simulink model "IceStorage_FHNW"  (R2018b)
settings: Solver=ode23  StartTime=-122*24*3600  StopTime=(365+181)*24*3600  EnableMultiTasking=on
StartFcn:
  | ticID_VsIceSTsim = tic;
StopFcn:
  | toc(ticID_VsIceSTsim)
undefined symbols (not defined in the file or in its folder): A, B, C, Davies, Dd, Hay
libraries: carnot x43, simulink x3, carsys x1
(part 1 of 2)
settings Model: SimulationMode=accelerator  Creator=ralf.dott  LastModifiedBy=drhf
settings DataIOCC: SaveFormat=Array  SignalLoggingSaveFormat=ModelDataLogs  SaveOutput=off  SignalLogging=off  DSMLogging=off  SaveTime=off
settings OptimizationCC: ExpressionDepthLimit=2147483647  LifeSpan=inf
settings DebuggingCC: UnderspecifiedInitializationDetection=Classic  MergeDetectMultiDrivingBlocksExec=none  SolverPrmCheckMsg=warning  FcnCallInpInsideContextMsg=warning  StateNameClashWarn=warning  SFUnexpectedBacktrackingDiag=warning  SFNoUnconditionalDefaultTransitionDiag=warning  SFExecutionAtInitializationDiag=none
settings HardwareCC: ProdBitPerPointer=32  ProdBitPerSizeT=32  ProdBitPerPtrDiffT=32  ProdLargestAtomicFloat=None  ProdIntDivRoundTo=Undefined  ProdEndianess=Unspecified  ProdWordSize=32  ProdHWDeviceType=32-bit Generic
settings ModelReferenceCC: PropagateSignalLabelsOutOfModel=off
settings SFSimCC: SimUseLocalCustomCode=off
settings RTWCC: RTWUseLocalCustomCode=off
settings CodeAppCC: StateflowObjectComments=on
settings GRTTargetCC: TargetLangStandard=C89/C90 (ANSI)  GeneratePreprocessorConditionals=Disable all  CombineOutputUpdateFcns=off  GRTInterface=on
settings ConfigComp: CovMetricSettings=dw  CovHtmlReporting=on  CovSaveCumulativeToWorkspaceVar=on  CovSaveSingleToWorkspaceVar=on  CovExternalEMLEnable=off

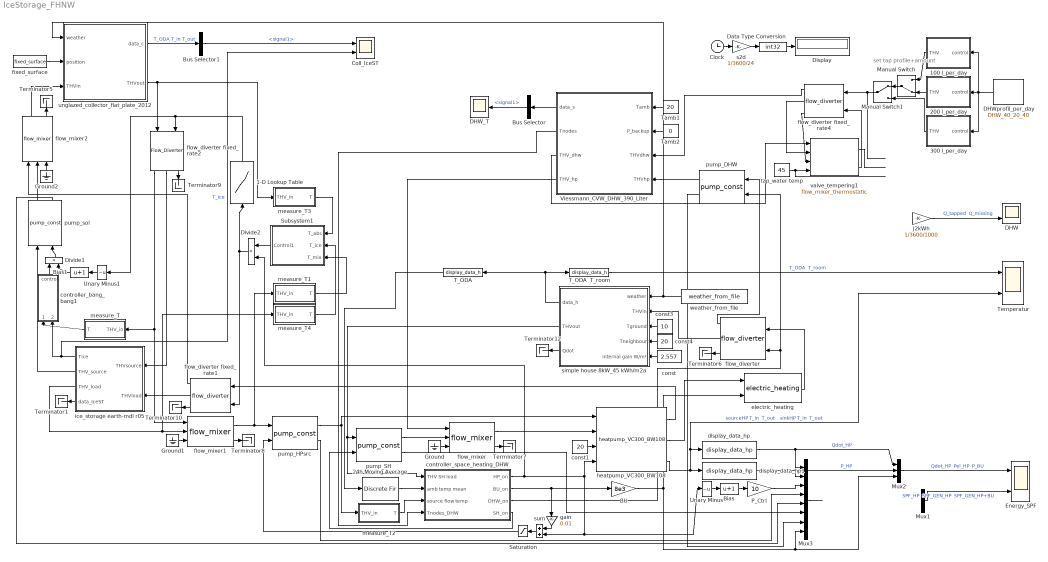
== system IceStorage_FHNW ==
  note: set tap
      | profile+amount
  1-D Lookup Table : Lookup_n-D  NumberOfTableDimensions=1  BreakpointsForDimension1=[-10, 0, eps, 10]  Table=[0, 0, 1, 1]  RndMeth=Simplest  InputSameDT=on
  100 l_per_day : Subsystem  mask(water tap){T=10, Tamp=3, dshift=-137, mdot=100/1800, fluid_id=water, mix=0, dia=0.013, p=2e5}
      mask prompts: T "mean temperature [degree centigrade]"; Tamp "amplitude of the sine [k]"; dshift "phase shift of the sine in [days]"; mdot "massflow [kg/s]"; fluid_id "fluid"; mix "percentage of fluid mix [0..1]"; dia "diameter at outlet [m]"; p "system pressure [Pa]"
      mask help:
      | The block models a tap, that produces a constant massflow of a fluid at given times.
      | control = 1 is full massflow, control = 0 is no massflow.
      | The temperature is a sine wave according to:
      |
      | T(out) = T(mean) + T(amplitude) * sin( 2*PI*(SimulationDay + DayPhaseShift) / 365 )
      mask init:
      | mdot = max(0, mdot);
      | mix = min(1, max(0, mix));
      | dia = max(0.001, dia);
      | p = max(p, 1e5);
      mask Help: eval('htmlhelp (''chap_4_2w.htm#water_tap'')')
      mask TypeOptions fluid_id: water | air | cotton_oil | silicone_oil | water_glycol_mix
      mask Display: plot(-10,10,90,90,[44,67,67,45,45,40,40,44],[80,80,72,72,60,60,76,80],[60,45],[90,90],[53,53],[80,90],[24,29,70,75,24],[30,10,10,30,30],[42,42],[32,58],[46,44],[34,54],[38,40],[34,56])
  200 l_per_day : Subsystem  mask(water tap){T=10, Tamp=3, dshift=-137, mdot=200/1800, fluid_id=water, mix=0, dia=0.013, p=2e5}
      mask prompts: T "mean temperature [degree centigrade]"; Tamp "amplitude of the sine [k]"; dshift "phase shift of the sine in [days]"; mdot "massflow [kg/s]"; fluid_id "fluid"; mix "percentage of fluid mix [0..1]"; dia "diameter at outlet [m]"; p "system pressure [Pa]"
      mask help:
      | The block models a tap, that produces a constant massflow of a fluid at given times.
      | control = 1 is full massflow, control = 0 is no massflow.
      | The temperature is a sine wave according to:
      |
      | T(out) = T(mean) + T(amplitude) * sin( 2*PI*(SimulationDay + DayPhaseShift) / 365 )
      mask init:
      | mdot = max(0, mdot);
      | mix = min(1, max(0, mix));
      | dia = max(0.001, dia);
      | p = max(p, 1e5);
      mask Help: eval('htmlhelp (''chap_4_2w.htm#water_tap'')')
      mask TypeOptions fluid_id: water | air | cotton_oil | silicone_oil | water_glycol_mix
      mask Display: plot(-10,10,90,90,[44,67,67,45,45,40,40,44],[80,80,72,72,60,60,76,80],[60,45],[90,90],[53,53],[80,90],[24,29,70,75,24],[30,10,10,30,30],[42,42],[32,58],[46,44],[34,54],[38,40],[34,56])
  24h Moving Average : DiscreteFir  Coefficients=ones(1,24)*(1/24)  SampleTime=3600  RndMeth=Nearest
  300 l_per_day : Subsystem  mask(water tap){T=10, Tamp=3, dshift=-137, mdot=300/1800, fluid_id=water, mix=0, dia=0.013, p=2e5}
      mask prompts: T "mean temperature [degree centigrade]"; Tamp "amplitude of the sine [k]"; dshift "phase shift of the sine in [days]"; mdot "massflow [kg/s]"; fluid_id "fluid"; mix "percentage of fluid mix [0..1]"; dia "diameter at outlet [m]"; p "system pressure [Pa]"
      mask help:
      | The block models a tap, that produces a constant massflow of a fluid at given times.
      | control = 1 is full massflow, control = 0 is no massflow.
      | The temperature is a sine wave according to:
      |
      | T(out) = T(mean) + T(amplitude) * sin( 2*PI*(SimulationDay + DayPhaseShift) / 365 )
      mask init:
      | mdot = max(0, mdot);
      | mix = min(1, max(0, mix));
      | dia = max(0.001, dia);
      | p = max(p, 1e5);
      mask Help: eval('htmlhelp (''chap_4_2w.htm#water_tap'')')
      mask TypeOptions fluid_id: water | air | cotton_oil | silicone_oil | water_glycol_mix
      mask Display: plot(-10,10,90,90,[44,67,67,45,45,40,40,44],[80,80,72,72,60,60,76,80],[60,45],[90,90],[53,53],[80,90],[24,29,70,75,24],[30,10,10,30,30],[42,42],[32,58],[46,44],[34,54],[38,40],[34,56])
  BU : Gain  Gain=8e3
  Bias : Bias  Bias=1
  Bias1 : Bias  Bias=1
  Bus Selector : BusSelector  OutputSignals=signal1
  Bus Selector1 : BusSelector  OutputSignals=signal1
  Clock : Clock
      settings: Decimation=3600
  Coll_IceST : Scope  NumInputPorts=2
  DHW : Scope  NumInputPorts=2
  DHW_T : Scope
  DHWprofil_per_day : carnot/loads/DHW_40_20_40  period=24*3600  rep_seq_t=[7 12 19]*3600  rep_seq_d=[0.2 0.1 0.2]*3600  rep_seq_y=[1 1 1]
      settings: SourceProductName=Carnot
  Data Type Conversion : DataTypeConversion  OutDataTypeStr=int32
  Display : Display
  Divide1 : Product  Inputs=**
  Divide2 : Product  Inputs=**
  Energy_SPF : Scope  NumInputPorts=2
  Ground : Ground
  Ground1 : Ground
  Ground2 : Ground
  J2kWh : Gain  Gain=1/3600/1000
  Manual Switch : ManualSwitch  CurrentSetting=0
  Manual Switch1 : ManualSwitch
  Mux1 : Mux  Inputs=3
  Mux2 : Mux  Inputs=3
  Mux3 : Mux  Inputs=8
  P_Ctrl : Gain  Gain=10
  Saturation : Saturate  UpperLimit=1  LowerLimit=0
  Subsystem1 : Subsystem
  T_ODA : carnot/outputs/display_data_h  a01=on  a02=off  a03=off  a04=off  a05=off  a06=off
      settings: SourceProductName=Carnot
  T_ODA  T_room : carnot/outputs/display_data_h  a01=on  a02=on  a03=off  a04=off  a05=off  a06=off
      settings: SourceProductName=Carnot
  Tamb1 : Constant  Value=20
  Tamb2 : Constant  Value=0
  Temperatur : Scope  NumInputPorts=2
  Terminator{1,5..10,12} (8 alike) : Terminator
  Unary Minus : UnaryMinus
  Unary Minus1 : UnaryMinus
  Viessmann_CVW_DHW_390_Liter : Subsystem  mask(storage with heat exchangers){diameter=0.65, vol=0.395, pos=standing cylinder, heatloss=2.34/(pi*0.65*(0.41/(pi*(0.65/2)^2))), hlossbot=0.34/(pi*(0.65/2)^2), hlosstop=2.34/(pi*0.65*(0.41/(pi*(0.65/2)^2))), axialcond=1.21, tinitial=45}
      mask prompts: diameter "diameter [m]"; vol "volume in [m³]"; pos "position"; heatloss "heat loss coefficient wall in [W/(m²*K)]"; hlossbot "heat loss coefficient bottom [W/(m²*K)]"; hlosstop "heat loss coefficient top [W/(m²*K)]"; axialcond "effective axial conductivity in [W/(m*K)]"; tinitial "initial temperature in [degree centigrade]"
      mask help:
      | Parameterized for the Vitocell 100-V type CVB, 300 liter domestic hot water cylinder.
      | Test data from itw 04STO103 06aug2004
      | Temperature sensor position (relative height)
      |     Solar: 0.04
      |     Backup heating DHW: 0.62
      mask Help: eval('man(''storage_multiport'')')
      mask TypeOptions pos: lying cylinder | standing cylinder
      mask Display: plot(0,0,100,100,[36,36,40,50,54,54,50,40,36],[90,50,45,45,50,90,93,93,90],[36,51,40,51,36],[74,74,79,85,85],[36,51,44,51,36],[54,54,56,58,58])
  const : Constant  Value=2.557
  const1 : Constant  Value=20
  const3 : Constant  Value=10
  const4 : Constant  Value=20
  controller_bang_bang1 : Subsystem  AncestorBlock=carnot/control/controller_bang_bang  mask(bang bang controler){deltaTon=6, deltaToff=2, Tmax=20}
      mask prompts: deltaTon "deltaT-on [K]"; deltaToff "deltaT-off [K]"; Tmax "maximum temperature Tcold [degree centigrade]"
      mask help:
      | Hysteresis controller for thermal systems. Output is set to zero if Thot or Tcold is bigger than Tmax.
      | deltaT = Thot - Tcold
      mask Help: eval('man (''bang_bang_controller'')')
      mask Display: plot(-30,0,150,100,[70,100,40,10,70,70,10,10],[50,80,80,50,50,20,20,50],[100,70],[50,20],[20,50,50,20,20],[40,40,30,30,40],[62,62,62,61,59,58,58,60],[42,41,39,38,38,40,42,43],[61,62,62,61,60,59,58,58,58,59],[32,31,30,28,27,28,28,30,31,32])
  controller_space_heating_DHW : Subsystem  mask(controller depending on ambient temperature and return temperature){Temin=-10, Ta_deltaHK=20, deltaHK=0, offsetTset=[0 0], HG=14, tmodi=[0 6 6 11 11 12 12 18 18 19 19 22 22 24]*3600, gammamodi=[1 1 1 1 1 1 1 1 0 0 1 1 1 1]*100   %100=spaceheating 200=DHW, deltaTRset=[1 -1], deltaTSset=[1 -1], Tiset=[20 20], tN=[22 6], m=1.1, TaD=-8, TD=[33 28], returnCTRLon=on, T_DHW=50, T_DHW_max=95, pos_DHW=0.4}
      mask prompts: Temin "min source input temperature [°C]"; Ta_deltaHK "ambient temperature for gradient modification [°C]"; deltaHK "elevation of feetpoint temperature [K] (for gradient modification)"; offsetTset "offset heating curve [TRset TSset]"; HG "heating limit"; tmodi "time values for schedule modi"; gammamodi "modi values for schedule modi"; deltaTRset "hysteresis TR lower and upper band [K]"; deltaTSset "hysteresis TS lower and upper band [K]"; Tiset "room temperature setpoint [day night] [°C]"; tN "night set back [starttime stoptime] [h]"; m "coefficient of heating surfaces [1...1.3]"; TaD "ambient temperature case of design [°C]"; TD "[supply return] temperature case of design [°C]"; returnCTRLon "control return temperature and connect return to "THV SH load" (off = flow temp.)"; T_DHW "domestic hot water temperature [°C]"; T_DHW_max "maximum domestic hot water temperature [°C]"; pos_DHW "storage height of control temp. sensor 0..1 (0=bottom 1=top)"
      mask help:
      | Calculating the heating curve dependent on return temperature and ambient temperature on basis of design temperature of return and supply as well as ambient design temperature with hysteresis.
      | The on SIA 384/2 based calculation of the heating curve can be modified to tune the gradient and give an offset.
      | With a time schedule the primacy of making warm water can be defined and a night set back can be destined.
      mask init:
      | if  tN(1)>24;
      |     error('unaccepted time values are set for night set back in block controller');
      | end;
      | if  tN(1)<0;
      |     error('unaccepted time values are set for night set back in block controller');
      | end;
      | if  tN(2)>24;
      |     error('unaccepted time values are set for night set back in block controller');
      | end;
      | if  tN(2)<0;
      |     error('unaccepted time values are set for night set back in block controller');
      | end;
      | if  m>2;
      |     error('unaccepted value for coefficient of heating surface in block controller');
      | end;
      | if  m>1.3;
      |     error('unaccepted value for coefficient of heating surface in block controller');
      | end;
      | if  m>1.3;
      |     error('unaccepted value for coefficient of heating surface in block controller');
      | end;
      | if  m<1;
      |     error('unaccepted value for coefficient of heating surface in block controller');
      | end;
      mask Help:
      | created   20.12.01 FHBB Institut of Energy suw
      | updated  18.01.02 FHBB Institut of Energy suw / night setback correction
      | updated  21.01.02 FHBB Institut of Energy suw / calculating TSset
      |                                                                            / using schedules
      |                                                                            / error criteria
      |                                                                            / heating limit HG
      |                                                                            / heating curve offset
      mask Display: plot(-100,-40,130,60, [70,10,70,70,10,10], [50,50,50,20,20,50], [20,50,50,20,20],[40,40,30,30,40], [62,62,62,61,59,58,58,60], [42,41,39,38,38,40,42,43], [61,62,62,61,60,59,58,58,58,59], [32,31,30,28,27,28,28,30,31,32])
  display_data_hp : carnot/outputs/display_data_hp  a1=off  a2=off  a3=off  a4=off  a5=off  a6=off  a7=off  a8=on  a9=off
      settings: SourceProductName=Carnot
  display_data_hp1 : carnot/outputs/display_data_hp  a1=off  a2=off  a3=off  a4=off  a5=off  a6=off  a7=off  a8=off  a9=on
      settings: SourceProductName=Carnot
  electric_heating : carnot/heat_source/electric_heating
      settings: SourceProductName=Carnot
  fixed_surface : carnot/weather/fixed_surface  colangle=40  colazi=0  colrot=0
      settings: SourceProductName=Carnot
  flow_diverter : carnot/hydraulics/flow_diverter  t=1
      settings: SourceProductName=Carnot
  flow_diverter fixed_rate1 : carnot/hydraulics/flow_diverter  t=5
      settings: SourceProductName=Carnot
  flow_diverter fixed_rate2 : carnot/hydraulics/Flow_Diverter  t=5
      settings: SourceProductName=Carnot
  flow_diverter fixed_rate4 : carnot/hydraulics/flow_diverter  t=5
      settings: SourceProductName=Carnot
  flow_mixer : carnot/hydraulics/flow_mixer  t=1
      settings: SourceProductName=Carnot
  flow_mixer1 : carnot/hydraulics/flow_mixer  t=1
      settings: SourceProductName=Carnot
  flow_mixer2 : carnot/hydraulics/flow_mixer  t=1
      settings: SourceProductName=Carnot
  gain : Gain  Gain=0.01
  heatpump_VC300_BW108 : carsys/heat_source/heatpump_VC300_BW108  caph=8*4e3  capc=4*4e3  dp=[100 1e4]  UA=5  Tcin=[0 15]  Thout=[35 55]  Qdoth=[7850 7100; 11500 10300]  Qdotc=[6300 4600; 9950 7850]  Pel=[1720 2690; 1670 2600]
      settings: SourceProductName=Carnot
  ice_storage earth-mdl r05 : Subsystem  mask(simple water storage){vol=10, l_solar=195, l_hp=7*50, f_ice=0, t_ini=15, z=3.32-0.12, h=2.3, dearth=0.5, Tmeanoutside=11, deltathetae=9.3, Tmeaninside=5, deltathetai=15, tshift=319, cond_ground=2, cp_ground=800, rho_ground=2500}
      mask prompts: vol "volume [m³]"; l_solar "length of solar heat exchanger [m]"; l_hp "length of HP heat exchanger [m]"; f_ice "Initial fraction of ice (0..1)"; t_ini "Initial Temperatur (only if fraction ice = 0) [°C]"; z "depth of baseplate from upper surface [m]"; h "height of ice storage [m]"; dearth "thickness of surrounding earth layer [m]"; Tmeanoutside "mean outside temperature over one year [°C]"; deltathetae "amplitude of monthly outside temperatures [°C]"; Tmeaninside "mean inside temperature over one year [°C]"; deltathetai "amplitude of monthly mean inside temperature [°C]"; tshift "time shift where external temperature sine-curve shows a minimum [h]"; cond_ground "conductivity of ground [W/(m*K)]"; cp_ground "capacity of ground [J/(kg*K)]"; rho_ground "density of ground [kg/m^3]"
      mask help: multinode water storage
      mask init:
      | f_ice = min(1, max(0, f_ice));
      | h_ini = (1-f_ice)*335e3;
      | if f_ice == 0 
      |     h_ini = h_ini + 4182*t_ini;
      | end
      | %Durchmesser Eisspeicher [m]
      | D_tank = 2.7;
      | %Höhe Eisspeicher [m]
      | h_tank = 2.3;
      | %Grundfläche [m^2]
      | A = pi*(D_tank/2.)^2;
      | %Umfang [m]
      | P = D_tank*pi;
      | %charakteristisches Bodenmass [m]
      | B = A/(0.5*P);
      | %Wärmewiderstand Boden & Wand [m^2*K/W]
      | Rbtot = 0.12/1.330;
      | Rwtot = 0.1/1.330;
      | %Wanddicke [m]
      | w = 0.1;
      | %wirksame Dicke Boden & Wand [m]
      | dt = w + cond_ground*Rbtot;
      | dw = cond_ground*Rwtot;
      | %abstand der mitte der wandfläche zur oberfläche [m]
      | ztilde = z-(0.5*h);
      | %anzahl stunden pro jahr
      | t0 = 8760;
      | %thermische eindringtiefe
      | delta_grd = sqrt((t0*3600*cond_ground)/(pi*rho_ground*cp_ground));
      | 
      | %U-Wert Erdschicht [W/m^2K]
      | U_earth = cond_ground/dearth;
      | %Oberfläche Erdschicht [m^2]
      | A_earth = ((D_tank+2*dearth)/2)^2*pi + (D_tank+2*dearth)*pi*(h_tank+dearth);
      | %Volumen Erdschicht [m^3]
      | V_earth = ((D_tank+2*dearth)/2)^2*pi*(h_tank+dearth) - (D_tank/2)^2*pi*h_tank;
      | %U*A tank
      | UA_tank = (D_tank/2)^2*pi/(0.12/1.330) + D_tank*pi*h_tank/(0.1/1.330);
      mask Help: eval('man(''storage'')')
      mask Display: plot(0,0,100,100,[20,30,40,50,60,70,70,60,50,40,30,20,20],[70,90,84,84,90,70,20,13,10,10,13,20,70],[60,50,40,30],[90,95,95,90],[70,60,50,40,30,20],[70,64,60,60,64,70],[45,45],[20,50],[56,35],[35,35],[53,37],[26,44],[53,37],[44,26],[48,45,42],[46,43,46],[54,51,54],[33,35,38],[48,45,42],[24,28,23],[37,40,37],[32,35,38])
  measure_T : Subsystem  mask(temperature measurement sensor){tc=300, t0=20}
      mask prompts: tc "time constant of sensor [s]"; t0 "initial temperature [degree centigrade]"
      mask help: Measurement sensor for temperatures with first-oder hold. Temperature is in degree centigrade.
      mask init:
      | tc = 1/max(tc, 0.001);
      mask Help: eval('man (''measure_T'')')
      mask Display: plot(-18,0,30,20,[0 20],[0 0],[10 10 8 8 12 12 10],[0 8 8 17 17 8 8],[10 10 9 9 11 11 10 9],[15 10 10 9 9 10 9 10])
  measure_T1 : Subsystem  mask(temperature measurement sensor){tc=300, t0=20}
      mask prompts: tc "time constant of sensor [s]"; t0 "initial temperature [degree centigrade]"
      mask help: Measurement sensor for temperatures with first-oder hold. Temperature is in degree centigrade.
      mask init:
      | tc = 1/max(tc, 0.001);
      mask Help: eval('man (''measure_T'')')
      mask Display: plot(-18,0,30,20,[0 20],[0 0],[10 10 8 8 12 12 10],[0 8 8 17 17 8 8],[10 10 9 9 11 11 10 9],[15 10 10 9 9 10 9 10])
  measure_T2 : Subsystem  mask(temperature measurement sensor){tc=300, t0=20}
      mask prompts: tc "time constant of sensor [s]"; t0 "initial temperature [degree centigrade]"
      mask help: Measurement sensor for temperatures with first-oder hold. Temperature is in degree centigrade.
      mask init:
      | tc = 1/max(tc, 0.001);
      mask Help: eval('man (''measure_T'')')
      mask Display: plot(-18,0,30,20,[0 20],[0 0],[10 10 8 8 12 12 10],[0 8 8 17 17 8 8],[10 10 9 9 11 11 10 9],[15 10 10 9 9 10 9 10])
  measure_T3 : Subsystem  mask(temperature measurement sensor){tc=300, t0=20}
      mask prompts: tc "time constant of sensor [s]"; t0 "initial temperature [degree centigrade]"
      mask help: Measurement sensor for temperatures with first-oder hold. Temperature is in degree centigrade.
      mask init:
      | tc = 1/max(tc, 0.001);
      mask Help: eval('man (''measure_T'')')
      mask Display: plot(-18,0,30,20,[0 20],[0 0],[10 10 8 8 12 12 10],[0 8 8 17 17 8 8],[10 10 9 9 11 11 10 9],[15 10 10 9 9 10 9 10])
  measure_T4 : Subsystem  mask(temperature measurement sensor){tc=300, t0=20}
      mask prompts: tc "time constant of sensor [s]"; t0 "initial temperature [degree centigrade]"
      mask help: Measurement sensor for temperatures with first-oder hold. Temperature is in degree centigrade.
      mask init:
      | tc = 1/max(tc, 0.001);
      mask Help: eval('man (''measure_T'')')
      mask Display: plot(-18,0,30,20,[0 20],[0 0],[10 10 8 8 12 12 10],[0 8 8 17 17 8 8],[10 10 9 9 11 11 10 9],[15 10 10 9 9 10 9 10])
  pump_DHW : carnot/hydraulics/pump_const  mdotmax=680/3600  fluid_id=water  mix=0  dia=0.402  power=34  p0=3e5  UA=0  tamb=20
      settings: SourceProductName=Carnot
  pump_HPsrc : carnot/hydraulics/pump_const  mdotmax=1160*1.050/3600  fluid_id=water_glycol_mix  mix=0.5  dia=0.402  power="49  % HX-ice + 2*25m + HX-HP at 1160L/h"  p0=3e5  UA=0  tamb=20
      settings: SourceProductName=Carnot
  pump_SH : carnot/hydraulics/pump_const  mdotmax=1360/3600  fluid_id=water  mix=0  dia=0.402  power=81  p0=3e5  UA=0  tamb=20
      settings: SourceProductName=Carnot
  pump_sol : carnot/hydraulics/pump_const  mdotmax=5*2.34*75/3600  fluid_id=water_glycol_mix  mix=0.5  dia=0.402  power=59 % 4*SLK-S + 2*40m + HXreg at 75l/m2/h  p0=3e5  UA=0  tamb=20
      settings: SourceProductName=Carnot
  s2d : Gain  Gain=1/3600/24
  simple house 8kW_45 kWh/m2a : Subsystem  AncestorBlock=carnot/loads/simple house  mask(simple house){Ahabit=250, Hroom=2.6, UA=[0.28*(97.6+47.2)+0.33*(69.4+70.0)*2  145*0.21*0.8  0], Awin=[12 4 3 4], AziWin=[0 90 -180 -90], Uwin=[1    1   1    1]*1., Gwin=[1    1   1    1]*0.595*(1-0.15), shade=0.75, tini=20, vent=0.7/2.6, rec=0, mc=0.5e6*250 % 0.5 MJ/m2/K, uaheating=5500/9, dpcoeff=[10 100]}
      mask prompts: Ahabit "ground surface in m²"; Hroom "height of rooms in m"; UA "heat transfer [to_ambient(walls/roof)  to_ground(floor)  to_neighbour] in W/K"; Awin "surface of 4 windows in m² (vector)"; AziWin "orientation of 4 windows (south 0, east -90,west 90)"; Uwin "heat loss coefficient 4 windows in W/m²/K [vector]"; Gwin "light transmittance 4 windows (0..1) * (1 - frame_part) [vector]"; shade "shading factor [0..1] when T room > 4 K + T_init"; tini "initial temperature"; vent "ventilation rate in 1/h"; rec "heat recovery (0..1)"; mc "total thermal capacity in J/K"; uaheating "heat transfer of the heating system in W/K"; dpcoeff "pressure drop coefficients [linear quadratic] in Pa/(kg/s), Pa/(kg/s)²"
      mask help:
      | Simple model of 1-node room or house. The differential equation
      | (m*c)house * dT/dt = solar_gain + internal_gain + heating_power - losses_to_ambient - losses_to_neighbour_room
      | is solved.
      | The heating power is generated by a radiator or floor heating system.
      | The windows have an automatic shading (shading factor) if room temperature rises 4 K above initial temperature.
      | solar gain = Solar_Radiation_on_window * light_transmittance * shading_factor
      | Use "look under mask" to set up the models parameters (initial conditions, surfaces characteristics...).
      | A usual value for the internal gains is 2.3 W/m².
      mask init:
      | invmc = 1/mc;
      | rec = max(0,min(1,rec));
      | Gwin = max(0,min(1,Gwin));
      | shade = max(0, min(1, shade));
      | UAout = UA(1);
      | UAground = UA(2);
      | UAin = UA(3);
      mask Help: eval('man(''simple_house'')')
      mask Display: plot(0,-15,80,100,[30,30,60,60,30],[20,50,50,20,20],[47,47,56,56,47],[40,30,30,40,40],[42,42,34,34],[20,40,40,20],[62,45,28],[48,70,48])
  sum : Sum  SaturateOnIntegerOverflow=on  InputSameDT=on  OutDataTypeStr=Inherit: Same as first input
  tap_water temp : Constant  Value=45
  unglazed_collector_flat_plate_2012 : Subsystem  AncestorBlock=carnot/new_blocks/unglazed_collector_flat_plate  mask(Unglazed flat plate collector){acol=5*2.544 %2.73, fta=0.978 %0.96, uc0=0, uc1=0, uc0loss=44.37 %45, uc1loss=8.62 %5, uc0gain=27.465 %35, uc1gain=47.14 %30, uc1eta0=0.021 %0.05, hi=165, e_sky=0.95, length=2.05, c_abs=38*1900/(2.34), c_fl=45*4187/(2.34), tini=15, nodes=5}
      mask prompts: acol "collector surface (aperture) in [m²]"; fta "absorption coefficient of the absorber [-]"; uc0 "linear heat transfer coefficient for condensation [W/(m²*K)]"; uc1 "wind dependent heat transfer coefficient for condensation [W/(m²*K*m/s)]"; uc0loss "linear heat transfer coefficient for convective loss [W/(m²*K)]"; uc1loss "wind dependent heat transfer coefficient for convective loss [W/(m²*K*m/s)]"; uc0gain "linear heat transfer coefficient for convective gains [W/(m²*K)]"; uc1gain "wind dependent heat transfer coefficient for convectiv gains [W/(m²*K*m/s)]"; uc1eta0 "wind denpendancy of optical efficiency in W/(m²*m/s)"; hi "heat transfer between collector and tube [W/(m2.K)]"; e_sky "emission coefficient of the absorber [-]"; length "length between inlet and outlet [m]"; c_abs "effective heat capacity of absorber [J/(m²*K)]"; c_fl "effective heat capacity of fluid [J/(m²*K)]"; tini "initial temperature [degree centigrade]"; nodes "number of nodes (>=2)"
      mask help:
      | 2xN-nodes model of an unglazed flat plate collector based on a model that includes
      | thermal capacity of the collector and the incidence angle modifier.
      | Look under mask to change the incidence angle modifier, the pressure drop and the radiation
      | calculation method.
      mask init:
      | %acol = max(acol, 0.01);
      | fta = max(fta,0);
      | c_abs = max(c_abs, 0.1);
      | 
      | %e_sky = 0.1;
      mask Help: eval('man(''collector_flat_plate'')')
      mask Display: plot(-10,0,80,78,[10 16 66 60 10],[16 10 60 66 16],[8,13],[8,13],[63,68],[63,68])
  valve_tempering1 : carnot/hydraulics/flow_mixer_thermostatic  t=300
      settings: SourceProductName=Carnot
  weather_from_file : carnot/weather/weather_from_file  file=DE_wuerzburg_3years  ext=.dat
      settings: SourceProductName=Carnot
  wires:
  weather_from_file/1 -> unglazed_collector_flat_plate_2012/1(weather), simple house 8kW_45 kWh/m2a/1(weather)
  const/1 -> simple house 8kW_45 kWh/m2a/5(internal gain W/m²)
  heatpump_VC300_BW108/2 -> electric_heating/1
  pump_HPsrc/1 -> measure_T2/1(THV_in), heatpump_VC300_BW108/1
  const1/1 -> heatpump_VC300_BW108/3
  simple house 8kW_45 kWh/m2a/2(THVout) -> controller_space_heating_DHW/1(THV SH load), pump_SH/1
  simple house 8kW_45 kWh/m2a/1(data_h) -> T_ODA  T_room/1, T_ODA/1
  T_ODA  T_room/1 -> Temperatur/1  "T_ODA  T_room"
  controller_space_heating_DHW/1(HP_on) -> Unary Minus/1, sum/2, heatpump_VC300_BW108/4, Divide2/2
  T_ODA/1 -> 24h Moving Average/1
  display_data_hp/1 -> Mux3/1, Mux2/1  "Qdot_HP"
  const3/1 -> simple house 8kW_45 kWh/m2a/3(Tground)
  24h Moving Average/1 -> controller_space_heating_DHW/2(amb temp mean)
  const4/1 -> simple house 8kW_45 kWh/m2a/4(Tneighbour)
  heatpump_VC300_BW108/1 -> flow_diverter fixed_rate1/1
  pump_SH/2 -> Mux3/6
  display_data_hp1/1 -> Mux3/2, Mux2/2  "P_HP"
  Mux2/1 -> Energy_SPF/1  "Qdot_HP  Pel_HP  P_BU"
  P_Ctrl/1 -> Mux3/3
  Mux3/1 -> ?
  tap_water temp/1 -> valve_tempering1/4
  valve_tempering1/2 -> flow_diverter fixed_rate4/2
  200 l_per_day/1(THV) -> Manual Switch/2
  valve_tempering1/1 -> ?
  DHWprofil_per_day/1 -> 200 l_per_day/1(control), 100 l_per_day/1(control), 300 l_per_day/1(control)
  flow_diverter fixed_rate4/3 -> valve_tempering1/3
  flow_diverter/1 -> pump_DHW/1
  pump_DHW/1 -> Viessmann_CVW_DHW_390_Liter/4(THVhp)
  pump_DHW/2 -> Mux3/7
  flow_diverter fixed_rate4/2 -> valve_tempering1/2
  100 l_per_day/1(THV) -> Manual Switch/1
  Manual Switch1/1 -> flow_diverter fixed_rate4/1
  Manual Switch/1 -> Manual Switch1/1
  300 l_per_day/1(THV) -> Manual Switch1/2
  Tamb1/1 -> Viessmann_CVW_DHW_390_Liter/1(Tamb)
  Viessmann_CVW_DHW_390_Liter/4(THV_hp) -> flow_mixer/1
  Viessmann_CVW_DHW_390_Liter/2(Tnodes) -> controller_space_heating_DHW/4(Tnodes_DHW)
  Viessmann_CVW_DHW_390_Liter/3(THV_dhw) -> valve_tempering1/1
  Viessmann_CVW_DHW_390_Liter/1(data_s) -> Bus Selector/1
  flow_diverter fixed_rate4/1 -> Viessmann_CVW_DHW_390_Liter/3(THVdhw)
  fixed_surface/1 -> unglazed_collector_flat_plate_2012/2(position)
  ice_storage earth-mdl r05/2(THV_source) -> pump_sol/1
  Tamb2/1 -> Viessmann_CVW_DHW_390_Liter/2(P_backup)
  flow_diverter/3 -> Terminator6/1
  flow_diverter/2 -> simple house 8kW_45 kWh/m2a/2(THVin)
  flow_mixer/1 -> heatpump_VC300_BW108/2
  pump_SH/1 -> flow_mixer/2
  flow_mixer/2 -> Terminator7/1
  unglazed_collector_flat_plate_2012/2(THVout) -> flow_diverter fixed_rate2/1, measure_T3/1(THV_in)
  Unary Minus/1 -> Bias/1
  Bias/1 -> P_Ctrl/1
  Ground/1 -> flow_mixer/3
  ice_storage earth-mdl r05/1(Tice) -> controller_bang_bang1/2(Tcold), Coll_IceST/2  "T_ice"
  pump_sol/1 -> flow_mixer2/2
  controller_bang_bang1/1(control) -> Divide1/1
  ? -> DHW/1  "T_cw  T_hw  T_DHWset"
  pump_HPsrc/2 -> Mux3/4
  pump_sol/2 -> Mux3/5
  heatpump_VC300_BW108/3 -> display_data_hp1/1, Temperatur/2, display_data_hp/1  "sourceHP T_in  T_out    sinkHP T_in  T_out"
  flow_mixer1/1 -> measure_T1/1(THV_in), pump_HPsrc/1
  flow_mixer1/2 -> Terminator8/1
  Ground1/1 -> flow_mixer1/3
  flow_diverter fixed_rate1/1 -> flow_mixer2/1
  flow_diverter fixed_rate1/2 -> ice_storage earth-mdl r05/2(THVload)
  ice_storage earth-mdl r05/3(THV_load) -> flow_mixer1/2, measure_T4/1(THV_in)
  Ground2/1 -> flow_mixer2/3
  flow_mixer2/2 -> Terminator5/1
  flow_diverter fixed_rate2/2 -> ice_storage earth-mdl r05/1(THVsource)
  flow_diverter fixed_rate2/1 -> flow_mixer1/1, measure_T/1(THV_in)
  flow_mixer2/1 -> unglazed_collector_flat_plate_2012/3(THVin)
  flow_diverter fixed_rate2/3 -> Terminator9/1
  flow_diverter fixed_rate1/3 -> Terminator10/1
  Unary Minus1/1 -> Bias1/1
  Bias1/1 -> Divide1/2
  Divide1/1 -> pump_sol/2
  measure_T/1(T) -> controller_bang_bang1/1(Thot)
  measure_T1/1(T) -> Subsystem1/3(T_mix)
  Divide2/1 -> flow_diverter fixed_rate1/2, 1-D Lookup Table/1
  unglazed_collector_flat_plate_2012/1(data_c) -> Bus Selector1/1  "T_ODA T_in T_out"
  simple house 8kW_45 kWh/m2a/3(Qdot) -> Terminator12/1
  ? -> J2kWh/1
  Mux1/1 -> Energy_SPF/2  "SPF_HP  SPF_GEN_HP  SPF_GEN_HP+BU"
  measure_T2/1(T) -> controller_space_heating_DHW/3(source flow temp)
  controller_space_heating_DHW/3(DHW_on) -> flow_diverter/2, pump_DHW/2
  controller_space_heating_DHW/4(SH_on) -> pump_SH/2
  electric_heating/1 -> flow_diverter/1
  controller_space_heating_DHW/2(BU_on) -> BU/1, gain/1
  BU/1 -> electric_heating/2, Mux3/8, Mux2/3
  sum/1 -> Saturation/1
  Saturation/1 -> pump_HPsrc/2
  gain/1 -> sum/1
  J2kWh/1 -> DHW/2  "Q_tapped  Q_missing"
  Clock/1 -> s2d/1
  s2d/1 -> Data Type Conversion/1
  Data Type Conversion/1 -> Display/1
  measure_T3/1(T) -> Subsystem1/1(T_abs)
  Subsystem1/1(Control1) -> Divide2/1
  measure_T4/1(T) -> Subsystem1/2(T_ice)
  1-D Lookup Table/1 -> Unary Minus1/1, flow_diverter fixed_rate2/2
  Bus Selector/1 -> DHW_T/1  "<signal1>"
  Bus Selector1/1 -> Coll_IceST/1  "<signal1>"
  ice_storage earth-mdl r05/4(data_IceST) -> Terminator1/1

== system IceStorage_FHNW/100 l_per_day ==
  control : Inport
  Ground : Ground
  ID1 : Constant
  Mux1 : Mux  Inputs=[1 1 1 7 10]
  Sine Wave : Sin  Amplitude=Tamp  Bias=T  Frequency=(2*pi/365/24/3600)  Phase=(2*pi*dshift/365)  SampleTime=0
  const1 : Constant  Value=[p fluid_id mix dia 0 0 0]
  mdot : Gain  Gain=mdot  SaturateOnIntegerOverflow=on  OutDataTypeStr=Inherit: Same as input  ParamDataTypeStr=Inherit: Same as input
  THV : Outport  InitialOutput=0
  wires:
  Sine Wave/1 -> Mux1/2
  ID1/1 -> Mux1/1
  Ground/1 -> Mux1/5
  const1/1 -> Mux1/4
  mdot/1 -> Mux1/3
  control/1 -> mdot/1
  Mux1/1 -> THV/1

== system IceStorage_FHNW/200 l_per_day ==
  control : Inport
  Ground : Ground
  ID1 : Constant
  Mux1 : Mux  Inputs=[1 1 1 7 10]
  Sine Wave : Sin  Amplitude=Tamp  Bias=T  Frequency=(2*pi/365/24/3600)  Phase=(2*pi*dshift/365)  SampleTime=0
  const1 : Constant  Value=[p fluid_id mix dia 0 0 0]
  mdot : Gain  Gain=mdot  SaturateOnIntegerOverflow=on  OutDataTypeStr=Inherit: Same as input  ParamDataTypeStr=Inherit: Same as input
  THV : Outport  InitialOutput=0
  wires:
  Mux1/1 -> THV/1
  control/1 -> mdot/1
  mdot/1 -> Mux1/3
  const1/1 -> Mux1/4
  Ground/1 -> Mux1/5
  ID1/1 -> Mux1/1
  Sine Wave/1 -> Mux1/2

== system IceStorage_FHNW/300 l_per_day ==
  control : Inport
  Ground : Ground
  ID1 : Constant
  Mux1 : Mux  Inputs=[1 1 1 7 10]
  Sine Wave : Sin  Amplitude=Tamp  Bias=T  Frequency=(2*pi/365/24/3600)  Phase=(2*pi*dshift/365)  SampleTime=0
  const1 : Constant  Value=[p fluid_id mix dia 0 0 0]
  mdot : Gain  Gain=mdot  SaturateOnIntegerOverflow=on  OutDataTypeStr=Inherit: Same as input  ParamDataTypeStr=Inherit: Same as input
  THV : Outport  InitialOutput=0
  wires:
  Mux1/1 -> THV/1
  control/1 -> mdot/1
  mdot/1 -> Mux1/3
  const1/1 -> Mux1/4
  Ground/1 -> Mux1/5
  ID1/1 -> Mux1/1
  Sine Wave/1 -> Mux1/2

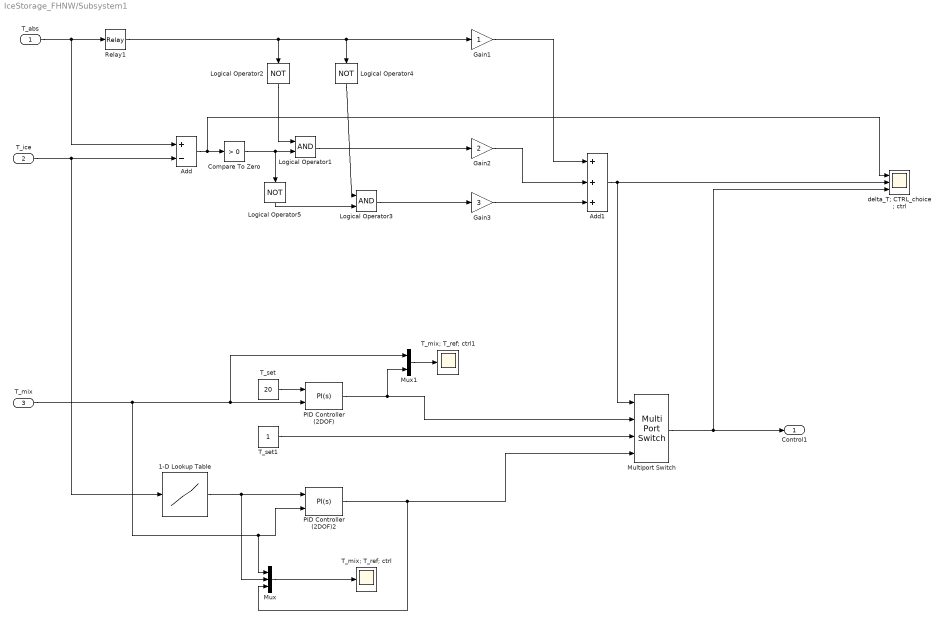
== system IceStorage_FHNW/Subsystem1 ==
  T_abs : Inport
  T_ice : Inport  Port=2
  T_mix : Inport  Port=3
  1-D Lookup Table : Lookup_n-D  NumberOfTableDimensions=1  BreakpointsForDimension1=[-10,-2:1:2,10]  Table=[-3,-3,-3,0,3,3,3]  RndMeth=Simplest  InputSameDT=on
  Add : Sum  Inputs=+-
  Add1 : Sum  Inputs=+++
  Compare To Zero : simulink/Logic and Bit Operations/Compare To Zero  relop=>  OutDataTypeStr=uint8
  Gain1 : Gain  ParamDataTypeStr=double
  Gain2 : Gain  Gain=2  ParamDataTypeStr=double
  Gain3 : Gain  Gain=3  ParamDataTypeStr=double
  Logical Operator1 : Logic  AllPortsSameDT=off  OutDataTypeStr=boolean
  Logical Operator2 : Logic  Operator=NOT  AllPortsSameDT=off  OutDataTypeStr=boolean
  Logical Operator3 : Logic  AllPortsSameDT=off  OutDataTypeStr=boolean
  Logical Operator4 : Logic  Operator=NOT  AllPortsSameDT=off  OutDataTypeStr=boolean
  Logical Operator5 : Logic  Operator=NOT  AllPortsSameDT=off  OutDataTypeStr=boolean
  Multiport Switch : MultiPortSwitch
  Mux : Mux  Inputs=3
  Mux1 : Mux  Inputs=2
  PID Controller (2DOF) : simulink/Continuous/PID Controller (2DOF)  Controller=PI  TimeDomain=Continuous-time  SampleTime=1  IntegratorMethod=Forward Euler  FilterMethod=Forward Euler  Form=Parallel  P=0  I=0.001  D=0  N=100  b=1  c=1  InitialConditionSource=internal  InitialConditionForIntegrator=0  InitialConditionForFilter=0  ExternalReset=none  LimitOutput=on  UpperSaturationLimit=1  LowerSaturationLimit=0  LinearizeAsGain=off  AntiWindupMode=clamping  Kb=1  TrackingMode=off  Kt=1  PParamMin=[]  PParamMax=[]  IParamMin=[]  IParamMax=[]  DParamMin=[]  DParamMax=[]  NParamMin=[]  NParamMax=[]  bParamMin=[]  bParamMax=[]  cParamMin=[]  cParamMax=[]  KbParamMin=[]  KbParamMax=[]  KtParamMin=[]  KtParamMax=[]  POutMin=[]  POutMax=[]  IOutMin=[]  IOutMax=[]  DOutMin=[]  DOutMax=[]  NOutMin=[]  NOutMax=[]  bOutMin=[]  bOutMax=[]  cOutMin=[]  cOutMax=[]  KbOutMin=[]  KbOutMax=[]  KtOutMin=[]  KtOutMax=[]  IntegratorOutMin=[]  IntegratorOutMax=[]  FilterOutMin=[]  FilterOutMax=[]  SumOutMin=[]  SumOutMax=[]  Sum1OutMin=[]  Sum1OutMax=[]  Sum2OutMin=[]  Sum2OutMax=[]  Sum3OutMin=[]  Sum3OutMax=[]  SumI1OutMin=[]  SumI1OutMax=[]  SumI2OutMin=[]  SumI2OutMax=[]  SumI3OutMin=[]  SumI3OutMax=[]  SumDOutMin=[]  SumDOutMax=[]  SaturationOutMin=[]  SaturationOutMax=[]  IntegratorContinuousStateAttributes=''  IntegratorStateMustResolveToSignalObject=off  IntegratorRTWStateStorageClass=Auto  FilterContinuousStateAttributes=''  FilterStateMustResolveToSignalObject=off  FilterRTWStateStorageClass=Auto
  PID Controller (2DOF)2 : simulink/Continuous/PID Controller (2DOF)  Controller=PI  TimeDomain=Continuous-time  SampleTime=1  IntegratorMethod=Forward Euler  FilterMethod=Forward Euler  Form=Parallel  P=0  I=-0.001  D=0  N=100  b=1  c=1  InitialConditionSource=internal  InitialConditionForIntegrator=0  InitialConditionForFilter=0  ExternalReset=none  LimitOutput=on  UpperSaturationLimit=1  LowerSaturationLimit=0  LinearizeAsGain=off  AntiWindupMode=clamping  Kb=1  TrackingMode=off  Kt=1  PParamMin=[]  PParamMax=[]  IParamMin=[]  IParamMax=[]  DParamMin=[]  DParamMax=[]  NParamMin=[]  NParamMax=[]  bParamMin=[]  bParamMax=[]  cParamMin=[]  cParamMax=[]  KbParamMin=[]  KbParamMax=[]  KtParamMin=[]  KtParamMax=[]  POutMin=[]  POutMax=[]  IOutMin=[]  IOutMax=[]  DOutMin=[]  DOutMax=[]  NOutMin=[]  NOutMax=[]  bOutMin=[]  bOutMax=[]  cOutMin=[]  cOutMax=[]  KbOutMin=[]  KbOutMax=[]  KtOutMin=[]  KtOutMax=[]  IntegratorOutMin=[]  IntegratorOutMax=[]  FilterOutMin=[]  FilterOutMax=[]  SumOutMin=[]  SumOutMax=[]  Sum1OutMin=[]  Sum1OutMax=[]  Sum2OutMin=[]  Sum2OutMax=[]  Sum3OutMin=[]  Sum3OutMax=[]  SumI1OutMin=[]  SumI1OutMax=[]  SumI2OutMin=[]  SumI2OutMax=[]  SumI3OutMin=[]  SumI3OutMax=[]  SumDOutMin=[]  SumDOutMax=[]  SaturationOutMin=[]  SaturationOutMax=[]  IntegratorContinuousStateAttributes=''  IntegratorStateMustResolveToSignalObject=off  IntegratorRTWStateStorageClass=Auto  FilterContinuousStateAttributes=''  FilterStateMustResolveToSignalObject=off  FilterRTWStateStorageClass=Auto
  Relay1 : Relay  OnSwitchValue=22  OffSwitchValue=20
  T_mix; T_ref; ctrl : Scope
  T_mix; T_ref; ctrl1 : Scope
  T_set : Constant  Value=20
  T_set1 : Constant
  delta_T; CTRL_choice ; ctrl : Scope  NumInputPorts=3
  Control1 : Outport
  wires:
  Mux/1 -> T_mix; T_ref; ctrl/1
  Logical Operator4/1 -> Logical Operator3/1
  Logical Operator5/1 -> Logical Operator3/2
  Logical Operator1/1 -> Gain2/1
  Logical Operator2/1 -> Logical Operator1/1
  1-D Lookup Table/1 -> Mux/2, PID Controller (2DOF)2/1
  Multiport Switch/1 -> Control1/1, delta_T; CTRL_choice ; ctrl/3
  PID Controller (2DOF)2/1 -> Mux/3, Multiport Switch/4
  Add1/1 -> Multiport Switch/1, delta_T; CTRL_choice ; ctrl/2
  Gain3/1 -> Add1/3
  Gain2/1 -> Add1/2
  Gain1/1 -> Add1/1
  T_set1/1 -> Multiport Switch/3
  Logical Operator3/1 -> Gain3/1
  Compare To Zero/1 -> Logical Operator5/1, Logical Operator1/2
  Add/1 -> delta_T; CTRL_choice ; ctrl/1, Compare To Zero/1
  T_ice/1 -> 1-D Lookup Table/1, Add/2
  PID Controller (2DOF)/1 -> Multiport Switch/2, Mux1/2
  T_set/1 -> PID Controller (2DOF)/1
  T_mix/1 -> Mux/1, PID Controller (2DOF)2/2, PID Controller (2DOF)/2, Mux1/1
  T_abs/1 -> Add/1, Relay1/1
  Mux1/1 -> T_mix; T_ref; ctrl1/1
  Relay1/1 -> Logical Operator4/1, Gain1/1, Logical Operator2/1

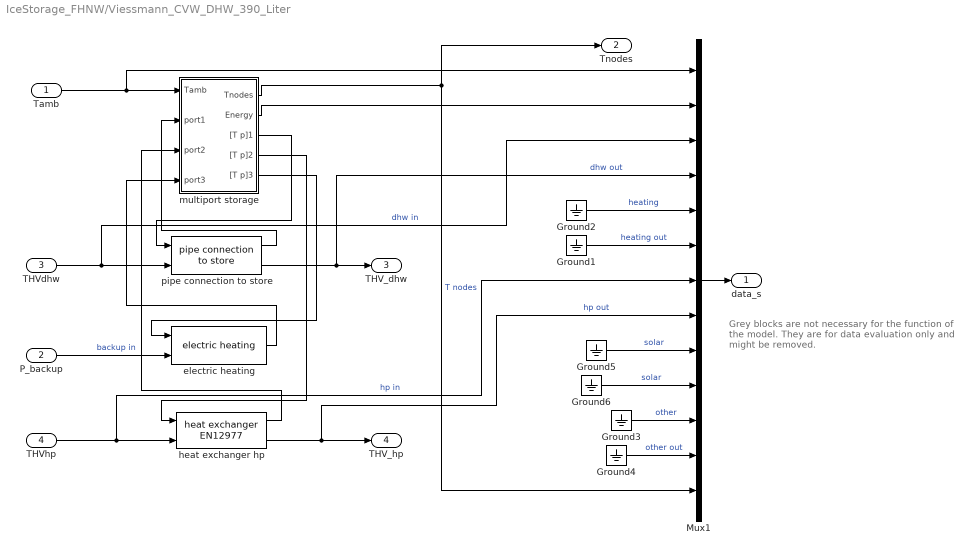
== system IceStorage_FHNW/Viessmann_CVW_DHW_390_Liter ==
  note: Grey blocks are not necessary for the function
      | of the model. They are for data evaluation only
      | and might be removed.
  Tamb : Inport
  P_backup : Inport  Port=2
  THVdhw : Inport  Port=3
  THVhp : Inport  Port=4
  Ground{1..6} (6 alike) : Ground
  Mux1 : Mux  Inputs=[1 14 20 20 20 20 20 20 20 20 20 20 -1]
  electric heating : carnot/storage/ports/electric heating  hin=0  hout=1
      settings: SourceProductName=Carnot
  heat exchanger hp : carnot/storage/ports/heat exchanger EN12977  hin=0.53  hout=0.07  ua0=350  uam=0.25  uat=0.5  dplin=100  dpqua=100
      settings: SourceProductName=Carnot
  multiport storage : Subsystem  mask(internal mask of storage for numerical values){nodes=84, sensors=21, nport=3, d=[diameter vol], u=[heatloss hlossbot hlosstop], axialcond=axialcond, tinitial=tinitial, pos=pos}
      mask prompts: nodes "number of nodes"; sensors "number of temperature sensors (first is at bottom)"; nport "number of ports"; d "geometry (DO NOT CHANGE HERE)"; u "heat losses (DO NOT CHANGE HERE)"; axialcond "effecive axial conductivity W/(m*K) (DO NOT CHANGE HERE)"; tinitial "initial temperature in °C (DO NOT CHANGE HERE)"; pos "position (DO NOT CHANGE HERE)"
      mask help: Model is one dimesional with <nodes> horizontal slices. Output sensor-temperatures are in equal distances over the storage (first output is lowest node).
      mask init:
      | nodes = max(nodes, 1);
      | sensors = max(sensors, 1);
      | d(1) = max(d(1), 0.001);
      | d(2) = max(d(2), 0.001);
      | pos = pos-1;
      mask Help:
      | The flow is calculated by the upwind scheme heat conduction between nodes by central diffenences (Patankar 1980).
      | Heat exchanger does not have any capacity for the fluid. Heat transfer to storage is calculated per stroage node by an energy balance. Heat transfer coefficient for heat exchanger is calculated from Nu = 0.5*(Gr*Pr)^0.25.
      | Can be charged and discharged by ports (straight incomming pipe, heat exchanger). For the moment You have to add the inports and outports yourself in  the subsystem when changing the number of ports. Be sure to keep the size of the demux after the s-funtion as [sensors 2  2  2] (repeat 2 as many ports as You have).
      mask TypeOptions nport: 1 | 2 | 3 | 4 | 5 | 6 | 7 | 8 | 9 | 10
  pipe connection to store : carnot/storage/ports/pipe connection to store  hin=0  hout=1
      settings: SourceProductName=Carnot
  data_s : Outport  InitialOutput=0
  Tnodes : Outport  Port=2  InitialOutput=0
  THV_dhw : Outport  Port=3  InitialOutput=0
  THV_hp : Outport  Port=4  InitialOutput=0
  wires:
  P_backup/1 -> electric heating/2  "backup in"
  THVhp/1 -> heat exchanger hp/2, Mux1/7  "hp in"
  heat exchanger hp/2 -> THV_hp/1, Mux1/8  "hp out"
  Tamb/1 -> multiport storage/1(Tamb), Mux1/1
  multiport storage/1(Tnodes) -> Mux1/13, Tnodes/1  "T nodes"
  multiport storage/3("[T p]1") -> pipe connection to store/1
  pipe connection to store/1 -> multiport storage/2(port1)
  multiport storage/4("[T p]2") -> heat exchanger hp/1
  heat exchanger hp/1 -> multiport storage/3(port2)
  multiport storage/5("[T p]3") -> electric heating/1
  electric heating/1 -> multiport storage/4(port3)
  Mux1/1 -> data_s/1
  pipe connection to store/2 -> Mux1/4, THV_dhw/1  "dhw out"
  THVdhw/1 -> pipe connection to store/2, Mux1/3  "dhw in"
  Ground2/1 -> Mux1/5  "heating"
  Ground1/1 -> Mux1/6  "heating out"
  Ground3/1 -> Mux1/11  "other"
  Ground4/1 -> Mux1/12  "other out"
  multiport storage/2(Energy) -> Mux1/2
  Ground5/1 -> Mux1/9  "solar"
  Ground6/1 -> Mux1/10  "solar"

== system IceStorage_FHNW/controller_bang_bang1 ==
  Thot : Inport
  Tcold : Inport  Port=2
  Constant : Constant  Value=Tmax
  Product : Product  OutDataTypeStr=double  SaturateOnIntegerOverflow=on
  Relational Operator : RelationalOperator  Operator=<=  RndMeth=Nearest  InputSameDT=on
  Relay : Relay  OnSwitchValue=deltaTon  OffSwitchValue=deltaToff
  Sum : Sum  Inputs=-+  SaturateOnIntegerOverflow=on  InputSameDT=on  OutDataTypeStr=Inherit: Same as first input
  control : Outport  InitialOutput=0
  wires:
  Relational Operator/1 -> Product/2
  Product/1 -> control/1
  Relay/1 -> Product/1
  Tcold/1 -> Sum/1, Relational Operator/1
  Thot/1 -> Sum/2
  Constant/1 -> Relational Operator/2
  Sum/1 -> Relay/1

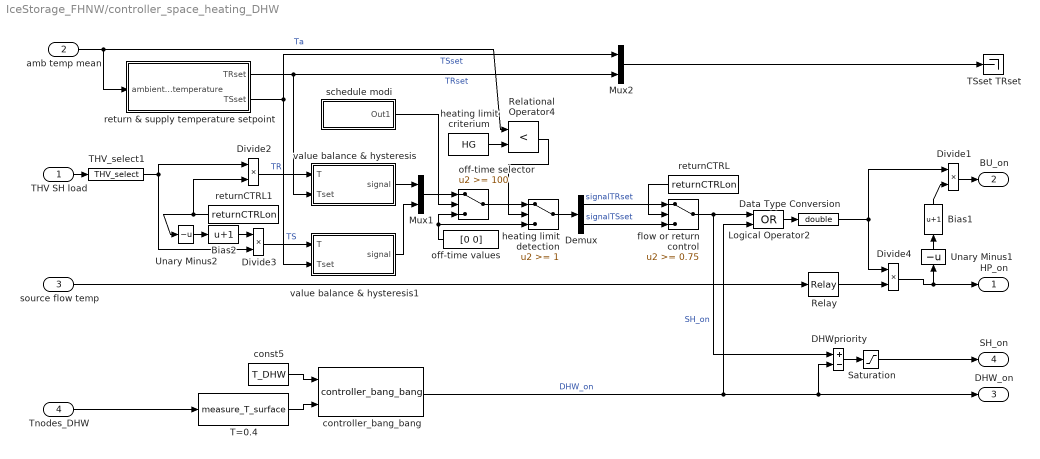
== system IceStorage_FHNW/controller_space_heating_DHW ==
  THV SH load : Inport
  amb temp mean : Inport  Port=2
  source flow temp : Inport  Port=3
  Tnodes_DHW : Inport  Port=4
  Bias1 : Bias  Bias=1
  Bias2 : Bias  Bias=1
  DHWpriority : Sum  Inputs=+-  SaturateOnIntegerOverflow=on  InputSameDT=on  OutDataTypeStr=Inherit: Same as first input
  Data Type Conversion : DataTypeConversion  OutDataTypeStr=double
  Demux : Demux  Outputs=2
  Divide{1..4} (4 alike) : Product  Inputs=**
  Logical Operator2 : Logic  Operator=OR  AllPortsSameDT=off
  Mux1 : Mux  Inputs=2
  Mux2 : Mux  Inputs=2
  Relational Operator4 : RelationalOperator  Operator=<  RndMeth=Nearest  InputSameDT=on
  Relay : Relay  OnSwitchValue=Temin+0.5  OffSwitchValue=Temin
  Saturation : Saturate  UpperLimit=1  LowerLimit=0
  T=0.4 : carnot/control/measure_T_surface  pos=pos_DHW  tdel=60  t0=20
      settings: SourceProductName=Carnot
  THV_select1 : carnot/outputs/THV_select  f=off  t=on  m=off  p=off  id=off  mix=off  d=off  dpcon=off  dplin=off  dpqua=off
      settings: SourceProductName=Carnot
  TSset TRset : Terminator
  Unary Minus1 : UnaryMinus
  Unary Minus2 : UnaryMinus
  const5 : Constant  Value=T_DHW
  controller_bang_bang : carnot/control/controller_bang_bang  deltaTon=5  deltaToff=0  Tmax=T_DHW_max
      settings: SourceProductName=Carnot
  flow or return control : Switch  Threshold=0.75  SaturateOnIntegerOverflow=on  InputSameDT=on
  heating limit criterium : Constant  Value=HG
  heating limit detection : Switch  Threshold=1  SaturateOnIntegerOverflow=on  InputSameDT=on
  off-time selector : Switch  Threshold=100  SaturateOnIntegerOverflow=on  InputSameDT=on
  off-time values : Constant  Value=[0 0]
  return & supply temperature setpoint : Subsystem
  returnCTRL : Constant  Value=returnCTRLon
  returnCTRL1 : Constant  Value=returnCTRLon
  schedule modi : Subsystem  mask(Repeating table){rep_seq_t=tmodi, rep_seq_y=gammamodi}
      mask prompts: rep_seq_t "Time values:"; rep_seq_y "Output values:"
      mask help: Output a repeating sequence of numbers specified in a table of time-value pairs. Values of time should be monotonically increasing.
      mask init:
      | if (length(rep_seq_t) ~= length(rep_seq_y)),
      |   error('Length of time vector and output vector must be the same.')
      | end
      | period = max(rep_seq_t) - min(rep_seq_t);
      | sim_start_time = eval(get_param(bdroot, 'StartTime'));
      | s = round(length(rep_seq_t)/50);
      | if s > 0
      |   disp_seq_t = rep_seq_t(1:s:end);
      |   disp_seq_y = rep_seq_y(1:s:end);
      |   disp_period = max(disp_seq_t) - min(disp_seq_t);
      | else
      |   disp_period = period;
      |   disp_seq_t = rep_seq_t;
      |   disp_seq_y = rep_seq_y;
      | end
      mask Help: Repeats cycle given in table. Time values should be monotonically increasing.
      mask Display:
      | plot( ...
      | [disp_seq_t, ...
      | disp_seq_t+disp_period, ...
      | disp_seq_t+2*disp_period, ...
      | disp_seq_t(1)+3*disp_period], ...
      | [disp_seq_y, ...
      | disp_seq_y, ...
      | disp_seq_y, ...
      | disp_seq_y(1)] ...
      | )
  value balance & hysteresis : Subsystem
  value balance & hysteresis1 : Subsystem
  HP_on : Outport
  BU_on : Outport  Port=2
  DHW_on : Outport  Port=3
  SH_on : Outport  Port=4
  wires:
  Saturation/1 -> SH_on/1
  Data Type Conversion/1 -> Divide1/1, Divide4/1
  DHWpriority/1 -> Saturation/1
  Logical Operator2/1 -> Data Type Conversion/1
  Bias2/1 -> Divide3/1
  returnCTRL1/1 -> Unary Minus2/1, Divide2/2
  THV_select1/1 -> Divide3/2, Divide2/1
  Divide2/1 -> value balance & hysteresis/1(T)  "TR"
  Unary Minus2/1 -> Bias2/1
  returnCTRL/1 -> flow or return control/2
  flow or return control/1 -> DHWpriority/1, Logical Operator2/1  "SH_on"
  controller_bang_bang/1 -> DHWpriority/2, DHW_on/1, Logical Operator2/2  "DHW_on"
  T=0.4/1 -> controller_bang_bang/2
  const5/1 -> controller_bang_bang/1
  Tnodes_DHW/1 -> T=0.4/1
  Mux2/1 -> TSset TRset/1
  Bias1/1 -> Divide1/2
  Divide1/1 -> BU_on/1
  Unary Minus1/1 -> Bias1/1
  Divide4/1 -> Unary Minus1/1, HP_on/1
  Divide3/1 -> value balance & hysteresis1/1(T)  "TS"
  THV SH load/1 -> THV_select1/1
  amb temp mean/1 -> Relational Operator4/1, return & supply temperature setpoint/1(ambient temperature)  "Ta"
  value balance & hysteresis/1(signal) -> Mux1/1
  value balance & hysteresis1/1(signal) -> Mux1/2
  off-time values/1 -> heating limit detection/3, off-time selector/3
  Mux1/1 -> off-time selector/1
  off-time selector/1 -> heating limit detection/1
  Demux/1 -> flow or return control/1  "signalTRset"
  Demux/2 -> flow or return control/3  "signalTSset"
  heating limit criterium/1 -> Relational Operator4/2
  Relational Operator4/1 -> heating limit detection/2
  heating limit detection/1 -> Demux/1
  return & supply temperature setpoint/2(TSset) -> Mux2/1, value balance & hysteresis1/2(Tset)  "TSset"
  return & supply temperature setpoint/1(TRset) -> Mux2/2, value balance & hysteresis/2(Tset)  "TRset"
  schedule modi/1(Out1) -> off-time selector/2
  source flow temp/1 -> Relay/1
  Relay/1 -> Divide4/2
